simulink model "Experiment_06081908_cs"  (R2021a)
settings: Solver=ode5  StartTime=0.0  StopTime=30  FixedStep=1/1000  RelTol=1e-3
PreLoadFcn:
  | mbxruntime.callbacks.PreLoadFcn(bdroot);
PostLoadFcn:
  | mbxruntime.callbacks.PostLoadFcn(bdroot);
InitFcn:
  | mbxruntime.callbacks.InitFcn(bdroot);
StartFcn:
  | mbxruntime.callbacks.StartFcn(bdroot);
StopFcn:
  | mbxruntime.callbacks.StopFcn(bdroot);
model workspace (MAT data in the model file):
  mbox_table : object (value not decoded)
  model_closed = 0
  sim_status = 0
values from neighbouring files (symbols this model uses):
  c_factor = 43.75    [emplanner_init.m]
  cf = -175016    [emplanner_init.m]
  cr = -130634    [emplanner_init.m]
  KD_PID_distance = 0.0    (= 0)    [emplanner_init.m]
  KD_PID_speed = 0    [emplanner_init.m]
  KI_PID_distance = 0.0    (= 0)    [emplanner_init.m]
  KI_PID_speed = 0    [emplanner_init.m]
  KP_PID_distance = 0.5    [emplanner_init.m]
  KP_PID_speed = 1.8    [emplanner_init.m]
  la = 1.265    [emplanner_init.m]
  lb = 2.947-1.265    (= 1.682)    [emplanner_init.m]
  LQR_K1 = k(:,1)'    [emplanner_init.m]
  LQR_K2 = k(:,2)'    [emplanner_init.m]
  LQR_K3 = k(:,3)'    [emplanner_init.m]
  LQR_K4 = k(:,4)'    [emplanner_init.m]
  m = 2020    [emplanner_init.m]
  rack_displacement = [-39.14 , -37.2 , -35.29 , -33.43 , -31.6 , -29.81 , -28.06 , -26.34 , -24.66 ,      -23.01 , -21.38 , -19.79 , -18.23 , -16.69 , -15.18 , -13.7 , -12.23 , -10.8 , -9.38 , -7.98 ,     -6.61 , -5.25 , -3.91 , -2.59 , -1.29 , 0 , 1.27 , 2.54 , 3.78 , 5.02 , 6.24 , 7.46 , 8.66 ,      9.86 , 11.05 , 12.24 , 13.41 , 14.59 , 15.76 , 16.92 , 18.09 , 19.25 , 20.42 , 21.59 , 22.76 ,      23.93 , 25.11 , 26 ...(+26 chars)    [emplanner_init.m]
  right_wheel_ground = [-70 ,-67.2 , -64.4 , -61.6 , -58.8 , -56 , -53.2 , -50.4 , -47.6 , -44.8 , -42 ,      -39.2 , -36.4 , -33.6 , -30.8 , -28 , -25.2 , -22.4 , -19.6 , -16.8 , -14 , -11.2 , -8.4 , -5.6 ,      -2.8 , 0 , 2.8 , 5.6 , 8.4 , 11.2 , 14 , 16.8 , 19.6 , 22.4 , 25.2 , 28 , 30.8 , 33.6 , 36.4 ,      39.2 , 42 , 44.8 , 47.6 , 50.4 , 53.2 , 56 , 58.8 , 61.6 , 64.4 , 67.2 , 70 ]    [emplanner_init.m]
  vx_break_point = zeros(1,5000)    [emplanner_init.m]
undefined symbols (not defined in the file or in its folder): aubr, DiscIntNeverNeededParam, global_path_x, global_path_y, tablebr, vubr
libraries: PreScanSimulinkLibrary x18, Solver_SF x1, simulink_extras x1
(part 4 of 8)

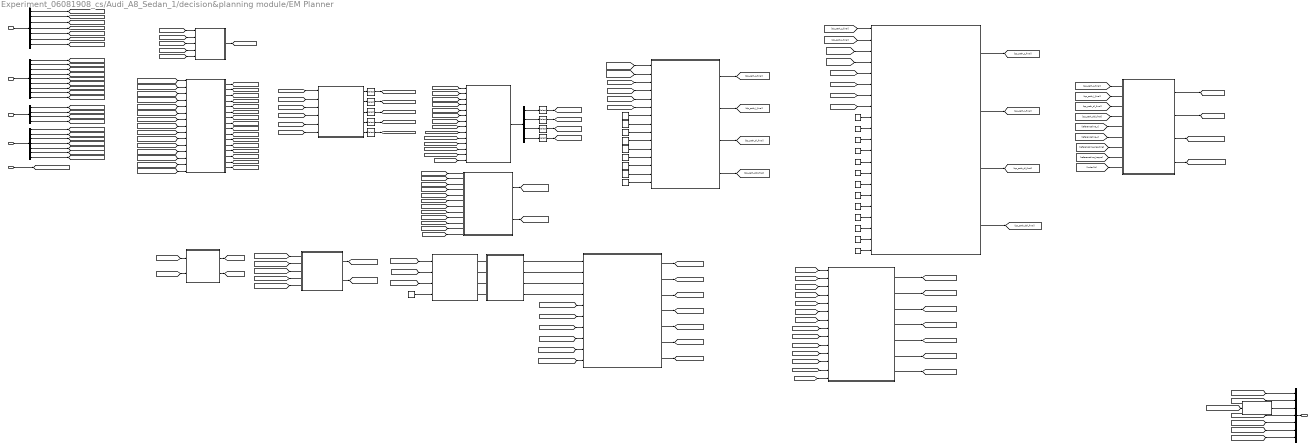
== system Experiment_06081908_cs/Audi_A8_Sedan_1/decision&planning module/EM Planner ==
  referenceline info : Inport
  location info : Inport  Port=2
  perception info : Inport  Port=3
  pre_planning info : Inport  Port=4
  current time : Inport  Port=5
  Bus Creator : BusCreator  Inputs=7
  Bus Selector : BusSelector  OutputSignals=referenceline_x,referenceline_y,referenceline_heading,referenceline_kappa,origin_match_point_index,origin_x,origin_y
  Bus Selector1 : BusSelector  OutputSignals=host_x,host_y,host_heading_xy,host_vx,host_vy,host_yawrate,host_speed,host_ax,host_ay
  Bus Selector2 : BusSelector  OutputSignals=obs_x_set_gcs,obs_y_set_gcs,obs_velocity_set_gcs,obs_heading_set_gcs
  Bus Selector3 : BusSelector  OutputSignals=trajectory_x_gcs,trajectory_y_gcs,trajectory_heading_gcs,trajectory_kappa_gcs,trajectory_speed_gcs,trajectory_accel_gcs,trajectory_time_gcs
  Bus Selector4 : BusSelector  OutputSignals=s_set,l_set,dl_set,ddl_set
  Cartesian2Frenet : Subsystem
  Constant : Constant  Value=1e6
  Constant1 : Constant  Value=2000
  Constant10 : Constant  Value=0.1
  Constant11 : Constant  Value=0.02
  Constant12 : Constant  Value=2
  Constant13 : Constant  Value=25000
  Constant14 : Constant  Value=50
  Constant15 : Constant  Value=20
  Constant{7,16..19} (5 alike) : Constant  Value=15
  Constant2 : Constant  Value=2
  Constant20 : Constant  Value=3
  Constant21 : Constant  Value=3
  Constant22 : Constant  Value=1.63
  Constant3 : Constant  Value=3
  Constant4 : Constant  Value=10
  Constant5 : Constant  Value=11
  Constant6 : Constant  Value=4
  Constant8 : Constant
  Constant9 : Constant  Value=6
  Frenet2Cartesian task : MATLAB Function  TreatAsAtomicUnit=on
  MATLAB Function : MATLAB Function  TreatAsAtomicUnit=on
  MATLAB Function2 : MATLAB Function  TreatAsAtomicUnit=on
  Selector{1..9} (9 alike) : Selector  InputPortWidth=128  IndexOptions=Index vector (dialog)  Indices=1  OutputSizes=1
  calc path length and map between point and s : MATLAB Function  TreatAsAtomicUnit=on
  calc plan start info and stitch trajectory : MATLAB Function  TreatAsAtomicUnit=on
  calc speed planning start condition : MATLAB Function  TreatAsAtomicUnit=on
  genrate index to s : MATLAB Function  TreatAsAtomicUnit=on
  increase st point count : MATLAB Function  TreatAsAtomicUnit=on
  obs : Subsystem
  path and speed merge : MATLAB Function  TreatAsAtomicUnit=on
  path decision task : Subsystem
  path planning task : Subsystem
  simple speed qp planning : MATLAB Function  TreatAsAtomicUnit=on
  stitch trajectory : MATLAB Function  TreatAsAtomicUnit=on
  EM Planner result : Outport
  wires:
  referenceline info/1 -> Bus Selector/1
  location info/1 -> Bus Selector1/1
  perception info/1 -> Bus Selector2/1
  pre_planning info/1 -> Bus Selector3/1
  current time/1 -> [current_time]
  Bus Selector3/1 -> [pre_trajectory_x_gcs]  "<trajectory_x_gcs>"
  Bus Selector3/2 -> [pre_trajectory_y_gcs]  "<trajectory_y_gcs>"
  Bus Selector3/3 -> [pre_trajectory_heading_gcs]  "<trajectory_heading_gcs>"
  Bus Selector3/4 -> [pre_trajectory_kappa_gcs]  "<trajectory_kappa_gcs>"
  Bus Selector3/5 -> [pre_trajectory_speed_gcs]  "<trajectory_speed_gcs>"
  Bus Selector3/6 -> [pre_trajectory_accel_gcs]  "<trajectory_accel_gcs>"
  Bus Selector3/7 -> [pre_trajectory_time]  "<trajectory_time_gcs>"
  Bus Selector2/1 -> [obs_x_set_gcs]  "<obs_x_set_gcs>"
  Bus Selector2/2 -> [obs_y_set_gcs]  "<obs_y_set_gcs>"
  Bus Selector2/3 -> [obs_velocity_set_gcs]  "<obs_velocity_set_gcs>"
  Bus Selector2/4 -> [obs_heading_set_gcs]  "<obs_heading_set_gcs>"
  Bus Selector1/1 -> [host_x]  "<host_x>"
  Bus Selector1/2 -> [host_y]  "<host_y>"
  Bus Selector1/3 -> [host_heading_xy]  "<host_heading_xy>"
  Bus Selector1/4 -> [host_vx_vcs]  "<host_vx>"
  Bus Selector1/5 -> [host_vy_vcs]  "<host_vy>"
  Bus Selector1/6 -> [host_yawrate]  "<host_yawrate>"
  Bus Selector1/7 -> [host_speed]  "<host_speed>"
  Bus Selector1/8 -> [host_ax_vcs]  "<host_ax>"
  Bus Selector1/9 -> [host_ay_vcs]  "<host_ay>"
  Bus Selector/1 -> [referenceline_x]  "<referenceline_x>"
  Bus Selector/2 -> [referenceline_y]  "<referenceline_y>"
  Bus Selector/3 -> [referenceline_heading]  "<referenceline_heading>"
  Bus Selector/4 -> [referenceline_kappa]  "<referenceline_kappa>"
  [host_ay_vcs] -> calc plan start info and stitch trajectory/15(host_ay)
  [host_ax_vcs] -> calc plan start info and stitch trajectory/14(host_ax)
  [host_vy_vcs] -> calc plan start info and stitch trajectory/13(host_vy)
  [host_vx_vcs] -> calc plan start info and stitch trajectory/12(host_vx)
  [host_heading_xy] -> calc plan start info and stitch trajectory/11(host_heading_xy)
  [host_y] -> calc plan start info and stitch trajectory/10(host_y)
  [host_x] -> calc plan start info and stitch trajectory/9(host_x)
  [current_time] -> calc plan start info and stitch trajectory/8(current_time)
  [pre_trajectory_x_gcs] -> calc plan start info and stitch trajectory/1(pre_trajectory_x)
  [pre_trajectory_y_gcs] -> calc plan start info and stitch trajectory/2(pre_trajectory_y)
  [pre_trajectory_time] -> calc plan start info and stitch trajectory/7(pre_trajectory_time)
  [pre_trajectory_accel_gcs] -> calc plan start info and stitch trajectory/6(pre_trajectory_accel)
  [pre_trajectory_speed_gcs] -> calc plan start info and stitch trajectory/5(pre_trajectory_velocity)
  [pre_trajectory_kappa_gcs] -> calc plan start info and stitch trajectory/4(pre_trajectory_kappa)
  [pre_trajectory_heading_gcs] -> calc plan start info and stitch trajectory/3(pre_trajectory_heading)
  calc plan start info and stitch trajectory/1(plan_start_x) -> [plan_start_x_gcs]
  calc plan start info and stitch trajectory/2(plan_start_y) -> [plan_start_y_gcs]
  calc plan start info and stitch trajectory/3(plan_start_heading) -> [plan_start_heading_gcs]
  calc plan start info and stitch trajectory/4(plan_start_kappa) -> [plan_start_kappa_gcs]
  calc plan start info and stitch trajectory/5(plan_start_vx) -> [plan_start_vx_gcs]
  calc plan start info and stitch trajectory/6(plan_start_vy) -> [plan_start_vy_gcs]
  calc plan start info and stitch trajectory/7(plan_start_ax) -> [plan_start_ax_gcs]
  calc plan start info and stitch trajectory/8(plan_start_ay) -> [plan_start_ay_gcs]
  calc plan start info and stitch trajectory/9(plan_start_time) -> [plan_start_time]
  calc plan start info and stitch trajectory/10(stitch_x) -> [stitch_x_gcs]
  calc plan start info and stitch trajectory/11(stitch_y) -> [stitch_y_gcs]
  calc plan start info and stitch trajectory/12(stitch_heading) -> [stitch_heading_gcs]
  calc plan start info and stitch trajectory/13(stitch_kappa) -> [stitch_kappa_gcs]
  calc plan start info and stitch trajectory/14(stitch_speed) -> [stitch_speed_gcs]
  calc plan start info and stitch trajectory/15(stitch_accel) -> [stitch_accel_gcs]
  calc plan start info and stitch trajectory/16(stitch_time) -> [stitch_time]
  Bus Selector/5 -> [origin_match_point_index]  "<origin_match_point_index>"
  Bus Selector/6 -> [origin_x]  "<origin_x>"
  Bus Selector/7 -> [origin_y]  "<origin_y>"
  [referenceline_x] -> genrate index to s/1(path_x)
  [referenceline_y] -> genrate index to s/2(path_y)
  [origin_x] -> genrate index to s/3(origin_x)
  [origin_y] -> genrate index to s/4(origin_y)
  [origin_match_point_index] -> genrate index to s/5(origin_match_point_index)
  genrate index to s/1(index2s) -> [index2s]
  MATLAB Function2/5(proj_kappa_set) -> Selector5/1
  MATLAB Function2/3(proj_y_set) -> Selector3/1
  MATLAB Function2/1(match_point_index_set) -> Selector1/1
  MATLAB Function2/4(proj_heading_set) -> Selector4/1
  MATLAB Function2/2(proj_x_set) -> Selector2/1
  [plan_start_x_gcs] -> MATLAB Function2/1(x_set)
  [plan_start_y_gcs] -> MATLAB Function2/2(y_set)
  [referenceline_x] -> MATLAB Function2/3(frenet_path_x)
  [referenceline_y] -> MATLAB Function2/4(frenet_path_y)
  [referenceline_heading] -> MATLAB Function2/5(frenet_path_heading)
  [referenceline_kappa] -> MATLAB Function2/6(frenet_path_kappa)
  Selector1/1 -> [plan_start_match_point_index]
  Selector2/1 -> [plan_start_proj_x]
  Selector3/1 -> [plan_start_proj_y]
  Selector4/1 -> [plan_start_proj_heading]
  Selector5/1 -> [plan_start_proj_kappa]
  [plan_start_y_gcs] -> Cartesian2Frenet/2(y_set)
  [plan_start_x_gcs] -> Cartesian2Frenet/1(x_set)
  [plan_start_vx_gcs] -> Cartesian2Frenet/3(vx_set)
  [plan_start_vy_gcs] -> Cartesian2Frenet/4(vy_set)
  [plan_start_ax_gcs] -> Cartesian2Frenet/5(ax_set)
  [plan_start_ay_gcs] -> Cartesian2Frenet/6(ay_set)
  [referenceline_x] -> Cartesian2Frenet/7(frenet_path_x)
  [referenceline_y] -> Cartesian2Frenet/8(frenet_path_y)
  [plan_start_match_point_index] -> Cartesian2Frenet/9(proj_match_point_index_set)
  [plan_start_proj_x] -> Cartesian2Frenet/10(proj_x_set)
  [plan_start_proj_y] -> Cartesian2Frenet/11(proj_y_set)
  [plan_start_proj_heading] -> Cartesian2Frenet/12(proj_heading_set)
  [plan_start_proj_kappa] -> Cartesian2Frenet/13(proj_kappa_set)
  Cartesian2Frenet/1(Cartesian2FrenetOut) -> Bus Selector4/1
  Bus Selector4/4 -> Selector9/1  "<ddl_set>"
  Bus Selector4/3 -> Selector8/1  "<dl_set>"
  Bus Selector4/2 -> Selector7/1  "<l_set>"
  Bus Selector4/1 -> Selector6/1  "<s_set>"
  Selector6/1 -> [plan_start_s]
  Selector7/1 -> [plan_start_l]
  Selector8/1 -> [plan_start_dl]
  Selector9/1 -> [plan_start_ddl]
  [index2s] -> Cartesian2Frenet/14(index2s)
  [host_x] -> obs/1(host_x)
  [host_y] -> obs/2(host_y)
  [host_heading_xy] -> obs/3(host_heading_xy)
  [obs_x_set_gcs] -> obs/4(obs_x_set_gcs)
  [obs_y_set_gcs] -> obs/5(obs_y_set_gcs)
  [obs_velocity_set_gcs] -> obs/6(obs_velocity_set_gcs)
  [obs_heading_set_gcs] -> obs/7(obs_heading_set_gcs)
  [referenceline_x] -> obs/8(referenceline_x)
  [referenceline_y] -> obs/9(referenceline_y)
  [referenceline_heading] -> obs/10(referenceline_heading)
  [referenceline_kappa] -> obs/11(referenceline_kappa)
  [index2s] -> obs/12(index2s)
  obs/1(static_obs_s_set) -> [static_obs_s_set]
  obs/2(static_obs_l_set) -> [static_obs_l_set]
  path and speed merge/7(trajectory_time) -> [trajectory_time]
  path and speed merge/1(trajectory_x) -> [trajectory_x]
  [trajectory_speed] -> stitch trajectory/5(trajectory_speed)
  path and speed merge/4(trajectory_kappa) -> [trajectory_kappa]
  [plan_start_vy_gcs] -> calc speed planning start condition/2(plan_start_vy)
  [stitch_time] -> stitch trajectory/14(stitch_time)
  calc path length and map between point and s/2(path_s) -> [path_s]
  [plan_start_heading_gcs] -> calc speed planning start condition/5(plan_start_heading)
  simple speed qp planning/2(s_dot_init) -> increase st point count/2(s_dot_init)
  Bus Creator/1 -> EM Planner result/1
  simple speed qp planning/1(s_init) -> increase st point count/1(s_init)
  [trajectory_x_final] -> Bus Creator/1  "trajectory_x_gcs"
  stitch trajectory/4(trajectory_kappa_final) -> [trajectory_kappa_final]
  [plan_start_ax_gcs] -> calc speed planning start condition/3(plan_start_ax)
  calc speed planning start condition/1(plan_start_s_dot) -> [plan_start_s_dot]
  [plan_start_ay_gcs] -> calc speed planning start condition/4(plan_start_ay)
  [stitch_speed_gcs] -> stitch trajectory/12(stitch_speed)
  [trajectory_time_final] -> Bus Creator/7  "trajectory_time_gcs"
  Constant9/1 -> simple speed qp planning/4(recommend_T)
  [stitch_x_gcs] -> stitch trajectory/8(stitch_x)
  stitch trajectory/1(trajectory_x_final) -> [trajectory_x_final]
  [trajectory_accel_final] -> Bus Creator/6  "trajectory_accel_gcs"
  [stitch_heading_gcs] -> stitch trajectory/10(stitch_heading)
  [trajectory_speed_final] -> Bus Creator/5  "trajectory_speed_gcs"
  [stitch_y_gcs] -> stitch trajectory/9(stitch_y)
  stitch trajectory/6(trajectory_accel_final) -> [trajectory_accel_final]
  [plan_start_s_dot2] -> simple speed qp planning/2(plan_start_s_dot2)
  increase st point count/3(s_dot2) -> path and speed merge/3(s_dot2)
  [plan_start_vx_gcs] -> calc speed planning start condition/1(plan_start_vx)
  [trajectory_heading_final] -> MATLAB Function/1(trajectory_heading_final)
  [trajectory_accel] -> stitch trajectory/6(trajectory_accel)
  [trajectory_kappa] -> stitch trajectory/4(trajectory_kappa)
  stitch trajectory/7(trajectory_time_final) -> [trajectory_time_final]
  [trajectory_x_init] -> path and speed merge/7(trajectory_x_init)
  stitch trajectory/2(trajectory_y_final) -> [trajectory_y_final]
  increase st point count/2(s_dot) -> path and speed merge/2(s_dot)
  stitch trajectory/3(trajectory_heading_final) -> [trajectory_heading_final]
  [trajectory_kappa_final] -> Bus Creator/4  "trajectory_kappa_gcs"
  [plan_start_s_dot] -> simple speed qp planning/1(plan_start_s_dot)
  path and speed merge/3(trajectory_heading) -> [trajectory_heading]
  simple speed qp planning/3(s_dot2_init) -> increase st point count/3(s_dot2_init)
  stitch trajectory/5(trajectory_speed_final) -> [trajectory_speed_final]
  [trajectory_y_final] -> Bus Creator/2  "trajectory_y_gcs"
  [trajectory_y] -> stitch trajectory/2(trajectory_y)
  calc path length and map between point and s/1(path_s_end) -> [path_s_end]
  calc speed planning start condition/2(plan_start_s_dot2) -> [plan_start_s_dot2]
  [trajectory_kappa_init] -> path and speed merge/10(trajectory_kappa_init)
  [stitch_accel_gcs] -> stitch trajectory/13(stitch_accel)
  increase st point count/1(s) -> path and speed merge/1(s)
  [trajectory_x] -> stitch trajectory/1(trajectory_x)
  [trajectory_y_init] -> calc path length and map between point and s/2(trajectory_y)
  [path_s_end] -> simple speed qp planning/3(s_end)
  path and speed merge/6(trajectory_accel) -> [trajectory_accel]
  [stitch_kappa_gcs] -> stitch trajectory/11(stitch_kappa)
  increase st point count/4(relative_time) -> path and speed merge/4(relative_time)
  [path_s] -> path and speed merge/6(path_s)
  path and speed merge/2(trajectory_y) -> [trajectory_y]
  [trajectory_heading_init] -> path and speed merge/9(trajectory_heading_init)
  [plan_start_time] -> path and speed merge/5(current_time)
  path and speed merge/5(trajectory_speed) -> [trajectory_speed]
  simple speed qp planning/4(relative_time_init) -> increase st point count/4(relative_time_init)
  [trajectory_y_init] -> path and speed merge/8(trajectory_y_init)
  [trajectory_time] -> stitch trajectory/7(trajectory_time)
  [trajectory_heading] -> stitch trajectory/3(trajectory_heading)
  [trajectory_x_init] -> calc path length and map between point and s/1(trajectory_x)
  [index2s] -> Frenet2Cartesian task/9(index2s)
  [referenceline_x] -> Frenet2Cartesian task/5(frenet_path_x)
  [referenceline_y] -> Frenet2Cartesian task/6(frenet_path_y)
  [referenceline_heading] -> Frenet2Cartesian task/7(frenet_path_heading)
  [referenceline_kappa] -> Frenet2Cartesian task/8(frenet_path_kappa)
  Frenet2Cartesian task/1(x_set) -> [trajectory_x_init]
  Frenet2Cartesian task/2(y_set) -> [trajectory_y_init]
  Frenet2Cartesian task/3(heading_set) -> [trajectory_heading_init]
  Frenet2Cartesian task/4(kappa_set) -> [trajectory_kappa_init]
  path decision task/1(dp_path_s_final) -> [dp_path_s_final]
  path decision task/2(dp_path_l_final) -> [dp_path_l_final]
  path decision task/3(dp_path_dl_final) -> [dp_path_dl_final]
  path decision task/4(dp_path_ddl_final) -> [dp_path_ddl_final]
  [static_obs_s_set] -> path decision task/1(static_obs_s_set)
  [static_obs_l_set] -> path decision task/2(static_obs_l_set)
  [plan_start_ddl] -> path decision task/6(plan_start_ddl)
  [plan_start_dl] -> path decision task/5(plan_start_dl)
  [plan_start_l] -> path decision task/4(plan_start_l)
  [plan_start_s] -> path decision task/3(plan_start_s)
  [dp_path_s_final] -> path planning task/1(dp_path_s_final)
  [dp_path_l_final] -> path planning task/2(dp_path_l_final)
  [plan_start_l] -> path planning task/6(plan_start_l)
  [plan_start_ddl] -> path planning task/8(plan_start_ddl)
  [plan_start_dl] -> path planning task/7(plan_start_dl)
  Constant22/1 -> path planning task/19(host_w)
  Constant21/1 -> path planning task/18(host_d2)
  Constant20/1 -> path planning task/17(host_d1)
  Constant19/1 -> path planning task/16(qp_cost_end_ddl)
  Constant18/1 -> path planning task/15(qp_cost_end_dl)
  Constant17/1 -> path planning task/14(qp_cost_endl)
  Constant16/1 -> path planning task/13(qp_cost_centre)
  Constant15/1 -> path planning task/12(qp_cost_dddl)
  Constant14/1 -> path planning task/11(qp_cost_ddl)
  Constant13/1 -> path planning task/10(qp_cost_dl)
  Constant12/1 -> path planning task/9(qp_cost_l)
  Constant8/1 -> path decision task/15(dp_sample_l)
  Constant7/1 -> path decision task/14(dp_sample_s)
  Constant6/1 -> path decision task/13(dp_col)
  Constant5/1 -> path decision task/12(dp_row)
  Constant4/1 -> path decision task/11(dp_cost_ref)
  Constant3/1 -> path decision task/10(dp_cost_dddl)
  Constant/1 -> path decision task/7(dp_cost_collision)
  Constant1/1 -> path decision task/8(dp_cost_dl)
  Constant2/1 -> path decision task/9(dp_cost_ddl)
  [static_obs_s_set] -> path planning task/3(static_obs_s_set)
  [static_obs_l_set] -> path planning task/4(static_obs_l_set)
  Constant10/1 -> path planning task/20(delta_dl_max)
  Constant11/1 -> path planning task/21(delta_ddl_max)
  path planning task/1(qp_path_s_final) -> [qp_path_s_final]
  path planning task/2(qp_path_l_final) -> [qp_path_l_final]
  path planning task/3(qp_path_dl_final) -> [qp_path_dl_final]
  path planning task/4(qp_path_ddl_final) -> [qp_path_ddl_final]
  [qp_path_ddl_final] -> Frenet2Cartesian task/4(ddl_set)
  [qp_path_l_final] -> Frenet2Cartesian task/2(l_set)
  [qp_path_dl_final] -> Frenet2Cartesian task/3(dl_set)
  [qp_path_s_final] -> Frenet2Cartesian task/1(s_set)
  [plan_start_s] -> path planning task/5(plan_start_s)
  MATLAB Function/1(y) -> Bus Creator/3  "trajectory_heading_gcs"

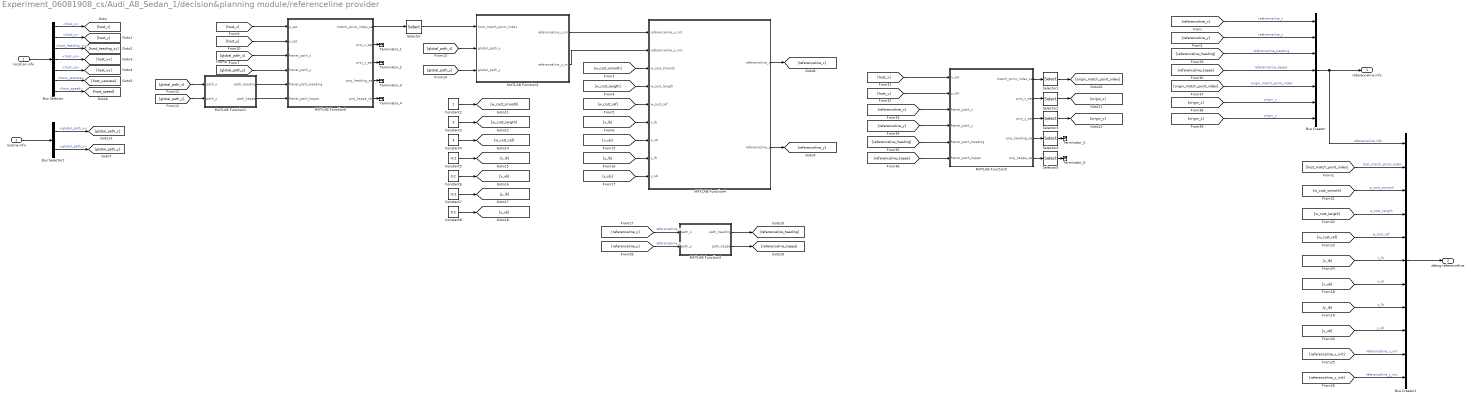
== system Experiment_06081908_cs/Audi_A8_Sedan_1/decision&planning module/referenceline provider ==
  location info : Inport
  routine info : Inport  Port=2
  Bus Creator : BusCreator  Inputs=7
  Bus Creator1 : BusCreator  Inputs=11
  Bus Selector : BusSelector  OutputSignals=host_x,host_y,host_heading_xy,host_vx,host_vy,host_yawrate,host_speed
  Bus Selector1 : BusSelector  OutputSignals=global_path_x,global_path_y
  Constant2 : Constant
  Constant3 : Constant  Value=2
  Constant4 : Constant  Value=3
  Constant5 : Constant  Value=-0.2
  Constant6 : Constant  Value=0.2
  Constant7 : Constant  Value=-0.2
  Constant8 : Constant  Value=0.2
  MATLAB Function1 : MATLAB Function  TreatAsAtomicUnit=on
  MATLAB Function2 : MATLAB Function  TreatAsAtomicUnit=on
  MATLAB Function3 : MATLAB Function  TreatAsAtomicUnit=on
  MATLAB Function4 : MATLAB Function  TreatAsAtomicUnit=on
  MATLAB Function5 : MATLAB Function  TreatAsAtomicUnit=on
  MATLAB Function6 : MATLAB Function  TreatAsAtomicUnit=on
  Selector{,1..5} (6 alike) : Selector  InputPortWidth=128  IndexOptions=Index vector (dialog)  Indices=1  OutputSizes=1
  Terminator_{1..6} (6 alike) : Terminator
  referenceline info : Outport
  debug referenceline : Outport  Port=2
  wires:
  [global_path_x] -> MATLAB Function2/2(global_path_x)
  [host_x] -> MATLAB Function6/1(x_set)
  MATLAB Function1/2(path_kappa) -> MATLAB Function6/6(frenet_path_kappa)
  MATLAB Function1/1(path_heading) -> MATLAB Function6/5(frenet_path_heading)
  [global_path_y] -> MATLAB Function6/4(frenet_path_y)
  [global_path_x] -> MATLAB Function6/3(frenet_path_x)
  [host_y] -> MATLAB Function6/2(y_set)
  [global_path_y] -> MATLAB Function1/2(path_y)
  [global_path_x] -> MATLAB Function1/1(path_x)
  Selector/1 -> MATLAB Function2/1(host_match_point_index)
  MATLAB Function6/1(match_point_index_set) -> Selector/1
  [global_path_y] -> MATLAB Function2/3(global_path_y)
  MATLAB Function2/1(referenceline_x_init) -> MATLAB Function4/1(referenceline_x_init)
  Bus Selector/5 -> [host_vy]  "<host_vy>"
  Bus Selector/1 -> [host_x]  "<host_x>"
  Bus Selector/2 -> [host_y]  "<host_y>"
  Bus Selector/3 -> [host_heading_xy]  "<host_heading_xy>"
  Bus Selector/4 -> [host_vx]  "<host_vx>"
  Bus Selector/7 -> [host_speed]  "<host_speed>"
  Bus Selector/6 -> [host_yawrate]  "<host_yawrate>"
  location info/1 -> Bus Selector/1
  Bus Selector1/2 -> [global_path_y]  "<global_path_y>"
  Bus Selector1/1 -> [global_path_x]  "<global_path_x>"
  routine info/1 -> Bus Selector1/1
  MATLAB Function4/1(referenceline_x) -> [referenceline_x]
  MATLAB Function4/2(referenceline_y) -> [referenceline_y]
  [referenceline_x] -> Bus Creator/1  "referenceline_x"
  [referenceline_y] -> Bus Creator/2  "referenceline_y"
  Bus Creator1/1 -> debug referenceline/1
  Bus Creator/1 -> Bus Creator1/1, referenceline info/1  "referenceline info"
  Constant2/1 -> [w_cost_smooth]
  Constant3/1 -> [w_cost_length]
  Constant8/1 -> [y_ub]
  Constant7/1 -> [y_lb]
  Constant6/1 -> [x_ub]
  Constant5/1 -> [x_lb]
  Constant4/1 -> [w_cost_ref]
  [w_cost_smooth] -> MATLAB Function4/3(w_cost_smooth)
  [w_cost_length] -> MATLAB Function4/4(w_cost_length)
  [w_cost_ref] -> MATLAB Function4/5(w_cost_ref)
  [x_lb] -> MATLAB Function4/6(x_lb)
  [x_ub] -> MATLAB Function4/7(x_ub)
  [y_lb] -> MATLAB Function4/8(y_lb)
  [y_ub] -> MATLAB Function4/9(y_ub)
  MATLAB Function2/2(referenceline_y_init) -> MATLAB Function4/2(referenceline_y_init)
  [w_cost_ref] -> Bus Creator1/5  "w_cost_ref"
  [x_lb] -> Bus Creator1/6  "x_lb"
  [w_cost_length] -> Bus Creator1/4  "w_cost_length"
  [x_ub] -> Bus Creator1/7  "x_ub"
  [w_cost_smooth] -> Bus Creator1/3  "w_cost_smooth"
  [y_lb] -> Bus Creator1/8  "y_lb"
  [host_match_point_index] -> Bus Creator1/2  "host_match_point_index"
  [y_ub] -> Bus Creator1/9  "y_ub"
  [referenceline_x_init] -> Bus Creator1/10  "referenceline_x_init"
  [referenceline_y_init] -> Bus Creator1/11  "referenceline_y_init"
  [referenceline_x] -> MATLAB Function3/1(path_x)  "referenceline_x"
  [referenceline_y] -> MATLAB Function3/2(path_y)  "referenceline_y"
  MATLAB Function3/1(path_heading) -> [referenceline_heading]
  MATLAB Function3/2(path_kappa) -> [referenceline_kappa]
  [referenceline_kappa] -> Bus Creator/4  "referenceline_kappa"
  [referenceline_heading] -> Bus Creator/3  "referenceline_heading"
  [host_x] -> MATLAB Function5/1(x_set)
  [host_y] -> MATLAB Function5/2(y_set)
  [referenceline_x] -> MATLAB Function5/3(frenet_path_x)
  [referenceline_y] -> MATLAB Function5/4(frenet_path_y)
  [referenceline_heading] -> MATLAB Function5/5(frenet_path_heading)
  [referenceline_kappa] -> MATLAB Function5/6(frenet_path_kappa)
  MATLAB Function5/1(match_point_index_set) -> Selector1/1
  MATLAB Function5/2(proj_x_set) -> Selector2/1
  MATLAB Function5/3(proj_y_set) -> Selector3/1
  MATLAB Function5/4(proj_heading_set) -> Selector4/1
  MATLAB Function5/5(proj_kappa_set) -> Selector5/1
  Selector1/1 -> [origin_match_point_index]
  Selector2/1 -> [origin_x]
  Selector3/1 -> [origin_y]
  [origin_match_point_index] -> Bus Creator/5  "origin_match_point_index"
  [origin_x] -> Bus Creator/6  "origin_x"
  [origin_y] -> Bus Creator/7  "origin_y"
  MATLAB Function6/2(proj_x_set) -> Terminator_1/1
  MATLAB Function6/3(proj_y_set) -> Terminator_2/1
  MATLAB Function6/4(proj_heading_set) -> Terminator_3/1
  MATLAB Function6/5(proj_kappa_set) -> Terminator_4/1
  Selector4/1 -> Terminator_5/1
  Selector5/1 -> Terminator_6/1

== system Experiment_06081908_cs/Audi_A8_Sedan_2/SELF_Demux/compas converter ==
  rotz [rad] : Inport
  cart2compas : Subsystem
  rad2deg : Gain  Gain=180/pi
  heading [deg] : Outport
  wires:
  rad2deg/1 -> cart2compas/1(Angle [deg])
  rotz [rad]/1 -> rad2deg/1
  cart2compas/1(heading [deg]) -> heading [deg]/1

== system Experiment_06081908_cs/Audi_A8_Sedan_2/Trajectories/Traj2State1 ==
  Traj Org : Inport
  Offset : Inport  Port=2
  Add2 : Sum
  ApplyRotation : PreScanSimulinkLibrary/ApplyRotation  SystemSampleTime=-1  VariantActivationTime=update diagram  Latency=0  AutoFrameSizeCalculation=off
  ApplyRotation1 : PreScanSimulinkLibrary/ApplyRotation  SystemSampleTime=-1  VariantActivationTime=update diagram  Latency=0  AutoFrameSizeCalculation=off
  ApplyRotation2 : PreScanSimulinkLibrary/ApplyRotation  SystemSampleTime=-1  VariantActivationTime=update diagram  Latency=0  AutoFrameSizeCalculation=off
  Constant : Constant  Value=zeros(12,1)
  Mux : Mux  Inputs=6
  Mux1 : Mux  Inputs=2
  Mux{2,4..9} (7 alike) : Mux  Inputs=3
  Mux3 : Mux  Inputs=2
  Selector : Selector  InputPortWidth=6  IndexOptions=Index vector (dialog)  Indices=[4 5 6]  OutputSizes=1
  Selector1 : Selector  InputPortWidth=21  IndexOptions=Index vector (dialog)  Indices=[5]  OutputSizes=1
  Selector10 : Selector  InputPortWidth=21  IndexOptions=Index vector (dialog)  Indices=[2]  OutputSizes=1
  Selector11 : Selector  InputPortWidth=21  IndexOptions=Index vector (dialog)  Indices=[3]  OutputSizes=1
  Selector12 : Selector  InputPortWidth=21  IndexOptions=Index vector (dialog)  Indices=[1]  OutputSizes=1
  Selector13 : Selector  InputPortWidth=21  IndexOptions=Index vector (dialog)  Indices=[8]  OutputSizes=1
  Selector14 : Selector  InputPortWidth=21  IndexOptions=Index vector (dialog)  Indices=[9]  OutputSizes=1
  Selector15 : Selector  InputPortWidth=21  IndexOptions=Index vector (dialog)  Indices=[7]  OutputSizes=1
  Selector16 : Selector  InputPortWidth=21  IndexOptions=Index vector (dialog)  Indices=[14]  OutputSizes=1
  Selector17 : Selector  InputPortWidth=21  IndexOptions=Index vector (dialog)  Indices=[15]  OutputSizes=1
  Selector18 : Selector  InputPortWidth=21  IndexOptions=Index vector (dialog)  Indices=[13]  OutputSizes=1
  Selector19 : Selector  InputPortWidth=21  IndexOptions=Index vector (dialog)  Indices=[20]  OutputSizes=1
  Selector2 : Selector  InputPortWidth=21  IndexOptions=Index vector (dialog)  Indices=[6]  OutputSizes=1
  Selector20 : Selector  InputPortWidth=21  IndexOptions=Index vector (dialog)  Indices=[21]  OutputSizes=1
  Selector21 : Selector  InputPortWidth=21  IndexOptions=Index vector (dialog)  Indices=[19]  OutputSizes=1
  Selector3 : Selector  InputPortWidth=21  IndexOptions=Index vector (dialog)  Indices=[12]  OutputSizes=1
  Selector4 : Selector  InputPortWidth=21  IndexOptions=Index vector (dialog)  Indices=[17]  OutputSizes=1
  Selector5 : Selector  InputPortWidth=21  IndexOptions=Index vector (dialog)  Indices=[18]  OutputSizes=1
  Selector6 : Selector  InputPortWidth=21  IndexOptions=Index vector (dialog)  Indices=[16]  OutputSizes=1
  Selector7 : Selector  InputPortWidth=21  IndexOptions=Index vector (dialog)  Indices=[11]  OutputSizes=1
  Selector8 : Selector  InputPortWidth=21  IndexOptions=Index vector (dialog)  Indices=[10]  OutputSizes=1
  Selector9 : Selector  InputPortWidth=21  IndexOptions=Index vector (dialog)  Indices=[4]  OutputSizes=1
  Traj2State2 : Subsystem
  state : Outport
  wires:
  Mux9/1 -> ApplyRotation2/2, ApplyRotation1/2, ApplyRotation/2
  Selector20/1 -> Mux9/3
  Selector19/1 -> Mux9/2
  Selector21/1 -> Mux9/1
  Selector5/1 -> Mux8/3
  Selector4/1 -> Mux8/2
  Selector6/1 -> Mux8/1
  Mux8/1 -> Mux/6
  Mux6/1 -> ApplyRotation2/1
  Mux7/1 -> Mux/4
  ApplyRotation2/1 -> Mux/5
  Selector3/1 -> Mux7/3
  Selector7/1 -> Mux7/2
  Selector8/1 -> Mux7/1
  Mux4/1 -> Mux/2
  Mux5/1 -> ApplyRotation1/1
  ApplyRotation1/1 -> Mux/3
  Mux2/1 -> ApplyRotation/1
  ApplyRotation/1 -> Mux/1
  Selector2/1 -> Mux4/3
  Selector1/1 -> Mux4/2
  Selector9/1 -> Mux4/1
  Selector17/1 -> Mux6/3
  Selector16/1 -> Mux6/2
  Selector18/1 -> Mux6/1
  Selector14/1 -> Mux5/3
  Selector13/1 -> Mux5/2
  Selector15/1 -> Mux5/1
  Selector11/1 -> Mux2/3
  Selector10/1 -> Mux2/2
  Selector12/1 -> Mux2/1
  Mux3/1 -> Selector8/1, Selector7/1, Selector3/1, Selector18/1, Selector16/1, Selector17/1, Selector6/1, Selector20/1, Selector19/1, Selector21/1, Selector5/1, Selector4/1, Selector14/1, Selector13/1, Selector15/1, Selector2/1, Selector1/1, Selector9/1, Selector12/1, Selector10/1, Selector11/1
  Mux1/1 -> Add2/2
  Constant/1 -> Mux1/2
  Add2/1 -> Traj2State2/1(traj)
  Selector/1 -> Mux3/2
  Traj Org/1 -> Mux3/1
  Offset/1 -> Mux1/1, Selector/1
  Mux/1 -> Add2/1
  Traj2State2/1(state) -> state/1

== system Experiment_06081908_cs/Audi_A8_Sedan_2/Trajectories/TrajCoGOffset ==
  State In : Inport
  Add : Sum  Inputs=+-+
  Add1 : Sum
  ApplyRotation : PreScanSimulinkLibrary/ApplyRotation  SystemSampleTime=-1  VariantActivationTime=update diagram  Latency=0  AutoFrameSizeCalculation=off
  ApplyRotation1 : PreScanSimulinkLibrary/ApplyRotation  SystemSampleTime=-1  VariantActivationTime=update diagram  Latency=0  AutoFrameSizeCalculation=off
  CoG Offset : Constant  Value=[0 0 CoGOffsetZ]
  Degrees to Radians : simulink_extras/Transformations/Degrees to Radians
  Demux1 : Demux  Outputs=[3 3 3]
  Mux : Mux  Inputs=[3 3 3]
  Orientation : Constant  Value=[InitRoll InitPitch 0]
  State Out : Outport
  wires:
  State In/1 -> Demux1/1
  Demux1/1 -> Add/1
  Add/1 -> Mux/1
  Demux1/3 -> Mux/3, Add1/2
  Mux/1 -> State Out/1
  Demux1/2 -> Mux/2
  Orientation/1 -> Degrees to Radians/1
  ApplyRotation/1 -> Add/3
  ApplyRotation1/1 -> Add/2
  Add1/1 -> ApplyRotation/2
  CoG Offset/1 -> ApplyRotation1/1, ApplyRotation/1
  Degrees to Radians/1 -> Add1/1, ApplyRotation1/2

== system Experiment_06081908_cs/Audi_A8_Sedan_2/Trajectories/Trajectory_1 ==
  From Workspace : FromWorkspace  VariableName=trajectory  SampleTime=TimeStep  ZeroCross=off  OutputAfterFinalValue=Holding final value
  From Workspace1 : FromWorkspace  VariableName=trajectory  SampleTime=TimeStep  ZeroCross=off  OutputAfterFinalValue=Setting to zero
  Mux : Mux  Inputs=2
  Selector1 : Selector  InputPortWidth=24  IndexOptions=Index vector (dialog)  Indices=[7:18]  OutputSizes=1
  Selector9 : Selector  InputPortWidth=24  IndexOptions=Index vector (dialog)  Indices=[1:6]  OutputSizes=1
  trajectory : Outport
  wires:
  From Workspace/1 -> Selector9/1
  From Workspace1/1 -> Selector1/1
  Mux/1 -> trajectory/1
  Selector9/1 -> Mux/1
  Selector1/1 -> Mux/2

== system Experiment_06081908_cs/Box_1/Dynamics_Empty/MuxState ==
  note: mode: Dynamics
  note: mode: Positioning
  note: mode: Dynamics
      | VelVEHICLE
      | wrt VEH
  note: AnglesVEHICLE
      | wrtGLOB
  note: For state mode 'Dynamic' positions
      | are not taken into account, as they
      | are computed by integrating velocity.
      | Click annotation for Help.
  x [m] : Inport  SampleTime=TimeStep
  y [m] : Inport  Port=2  SampleTime=TimeStep
  z [m] : Inport  Port=3  SampleTime=TimeStep
  dx [m/s] : Inport  Port=4  SampleTime=TimeStep
  dy [m/s] : Inport  Port=5  SampleTime=TimeStep
  dz [m/s] : Inport  Port=6  SampleTime=TimeStep
  R [rad] : Inport  Port=7  SampleTime=TimeStep
  P [rad] : Inport  Port=8  SampleTime=TimeStep
  Y [rad] : Inport  Port=9  SampleTime=TimeStep
  Constant : Constant  DisableCoverage=on  Value=positioningmode
  Discrete-Time Integrator : DiscreteIntegrator  SampleTime=TimeStep  ICPrevOutput=DiscIntNeverNeededParam  ICPrevScaledInput=DiscIntNeverNeededParam
  Ground : Ground
  Ground1 : Ground
  Mux1 : Mux  Inputs=[3 3]
  Mux2 : Mux  Inputs=3
  Mux3 : Mux  Inputs=3
  Mux4 : Mux  Inputs=3
  Mux5 : Mux  Inputs=[3 3]
  Mux6 : Mux  Inputs=[6 3]
  Switch : Switch  Threshold=0.5
  Transformation_BODY2GLOBAL : PreScanSimulinkLibrary/Simple_Vehicle_Dynamics/Chassis/MuxDynState/Transformation_BODY2GLOBAL  SystemSampleTime=-1  VariantActivationTime=update diagram  Latency=0  AutoFrameSizeCalculation=off
  mux3 : Mux  Inputs=3
  state : Outport
  wires:
  Constant/1 -> Switch/2
  Mux6/1 -> state/1
  Mux4/1 -> Mux1/1
  Mux5/1 -> Switch/3
  Mux1/1 -> Switch/1
  Switch/1 -> Mux6/1  "PosVeh wrt  GLOB"
  P [rad]/1 -> Mux3/2
  R [rad]/1 -> Mux3/1
  dz [m/s]/1 -> Mux2/3
  dy [m/s]/1 -> Mux2/2
  dx [m/s]/1 -> Mux2/1
  z [m]/1 -> Mux4/3
  y [m]/1 -> Mux4/2
  x [m]/1 -> Mux4/1
  Ground1/1 -> mux3/2  "pitch"
  Y [rad]/1 -> mux3/3, Mux3/3  "yaw"
  Mux3/1 -> Mux6/2
  Transformation_BODY2GLOBAL/1 -> Discrete-Time Integrator/1, Mux5/2  "VelVEH wrt  GLOB"
  mux3/1 -> Transformation_BODY2GLOBAL/2
  Ground/1 -> mux3/1  "roll"
  Mux2/1 -> Mux1/2, Transformation_BODY2GLOBAL/1
  Discrete-Time Integrator/1 -> Mux5/1  "PosVEH wrt  GLOB"

== system Experiment_06081908_cs/Box_1/SELF_Demux/compas converter ==
  rotz [rad] : Inport
  cart2compas : Subsystem
  rad2deg : Gain  Gain=180/pi
  heading [deg] : Outport
  wires:
  rad2deg/1 -> cart2compas/1(Angle [deg])
  rotz [rad]/1 -> rad2deg/1
  cart2compas/1(heading [deg]) -> heading [deg]/1

== system Experiment_06081908_cs/Box_2/Dynamics_Empty/MuxState ==
  note: mode: Dynamics
  note: mode: Positioning
  note: mode: Dynamics
      | VelVEHICLE
      | wrt VEH
  note: AnglesVEHICLE
      | wrtGLOB
  note: For state mode 'Dynamic' positions
      | are not taken into account, as they
      | are computed by integrating velocity.
      | Click annotation for Help.
  x [m] : Inport  SampleTime=TimeStep
  y [m] : Inport  Port=2  SampleTime=TimeStep
  z [m] : Inport  Port=3  SampleTime=TimeStep
  dx [m/s] : Inport  Port=4  SampleTime=TimeStep
  dy [m/s] : Inport  Port=5  SampleTime=TimeStep
  dz [m/s] : Inport  Port=6  SampleTime=TimeStep
  R [rad] : Inport  Port=7  SampleTime=TimeStep
  P [rad] : Inport  Port=8  SampleTime=TimeStep
  Y [rad] : Inport  Port=9  SampleTime=TimeStep
  Constant : Constant  DisableCoverage=on  Value=positioningmode
  Discrete-Time Integrator : DiscreteIntegrator  SampleTime=TimeStep  ICPrevOutput=DiscIntNeverNeededParam  ICPrevScaledInput=DiscIntNeverNeededParam
  Ground : Ground
  Ground1 : Ground
  Mux1 : Mux  Inputs=[3 3]
  Mux2 : Mux  Inputs=3
  Mux3 : Mux  Inputs=3
  Mux4 : Mux  Inputs=3
  Mux5 : Mux  Inputs=[3 3]
  Mux6 : Mux  Inputs=[6 3]
  Switch : Switch  Threshold=0.5
  Transformation_BODY2GLOBAL : PreScanSimulinkLibrary/Simple_Vehicle_Dynamics/Chassis/MuxDynState/Transformation_BODY2GLOBAL  SystemSampleTime=-1  VariantActivationTime=update diagram  Latency=0  AutoFrameSizeCalculation=off
  mux3 : Mux  Inputs=3
  state : Outport
  wires:
  Constant/1 -> Switch/2
  Mux6/1 -> state/1
  Mux4/1 -> Mux1/1
  Mux5/1 -> Switch/3
  Mux1/1 -> Switch/1
  Switch/1 -> Mux6/1  "PosVeh wrt  GLOB"
  P [rad]/1 -> Mux3/2
  R [rad]/1 -> Mux3/1
  dz [m/s]/1 -> Mux2/3
  dy [m/s]/1 -> Mux2/2
  dx [m/s]/1 -> Mux2/1
  z [m]/1 -> Mux4/3
  y [m]/1 -> Mux4/2
  x [m]/1 -> Mux4/1
  Ground1/1 -> mux3/2  "pitch"
  Y [rad]/1 -> mux3/3, Mux3/3  "yaw"
  Mux3/1 -> Mux6/2
  Transformation_BODY2GLOBAL/1 -> Discrete-Time Integrator/1, Mux5/2  "VelVEH wrt  GLOB"
  mux3/1 -> Transformation_BODY2GLOBAL/2
  Ground/1 -> mux3/1  "roll"
  Mux2/1 -> Mux1/2, Transformation_BODY2GLOBAL/1
  Discrete-Time Integrator/1 -> Mux5/1  "PosVEH wrt  GLOB"

== system Experiment_06081908_cs/Box_2/SELF_Demux/compas converter ==
  rotz [rad] : Inport
  cart2compas : Subsystem
  rad2deg : Gain  Gain=180/pi
  heading [deg] : Outport
  wires:
  rad2deg/1 -> cart2compas/1(Angle [deg])
  rotz [rad]/1 -> rad2deg/1
  cart2compas/1(heading [deg]) -> heading [deg]/1

== system Experiment_06081908_cs/Box_3/Dynamics_Empty/MuxState ==
  note: mode: Dynamics
  note: mode: Positioning
  note: mode: Dynamics
      | VelVEHICLE
      | wrt VEH
  note: AnglesVEHICLE
      | wrtGLOB
  note: For state mode 'Dynamic' positions
      | are not taken into account, as they
      | are computed by integrating velocity.
      | Click annotation for Help.
  x [m] : Inport  SampleTime=TimeStep
  y [m] : Inport  Port=2  SampleTime=TimeStep
  z [m] : Inport  Port=3  SampleTime=TimeStep
  dx [m/s] : Inport  Port=4  SampleTime=TimeStep
  dy [m/s] : Inport  Port=5  SampleTime=TimeStep
  dz [m/s] : Inport  Port=6  SampleTime=TimeStep
  R [rad] : Inport  Port=7  SampleTime=TimeStep
  P [rad] : Inport  Port=8  SampleTime=TimeStep
  Y [rad] : Inport  Port=9  SampleTime=TimeStep
  Constant : Constant  DisableCoverage=on  Value=positioningmode
  Discrete-Time Integrator : DiscreteIntegrator  SampleTime=TimeStep  ICPrevOutput=DiscIntNeverNeededParam  ICPrevScaledInput=DiscIntNeverNeededParam
  Ground : Ground
  Ground1 : Ground
  Mux1 : Mux  Inputs=[3 3]
  Mux2 : Mux  Inputs=3
  Mux3 : Mux  Inputs=3
  Mux4 : Mux  Inputs=3
  Mux5 : Mux  Inputs=[3 3]
  Mux6 : Mux  Inputs=[6 3]
  Switch : Switch  Threshold=0.5
  Transformation_BODY2GLOBAL : PreScanSimulinkLibrary/Simple_Vehicle_Dynamics/Chassis/MuxDynState/Transformation_BODY2GLOBAL  SystemSampleTime=-1  VariantActivationTime=update diagram  Latency=0  AutoFrameSizeCalculation=off
  mux3 : Mux  Inputs=3
  state : Outport
  wires:
  Constant/1 -> Switch/2
  Mux6/1 -> state/1
  Mux4/1 -> Mux1/1
  Mux5/1 -> Switch/3
  Mux1/1 -> Switch/1
  Switch/1 -> Mux6/1  "PosVeh wrt  GLOB"
  P [rad]/1 -> Mux3/2
  R [rad]/1 -> Mux3/1
  dz [m/s]/1 -> Mux2/3
  dy [m/s]/1 -> Mux2/2
  dx [m/s]/1 -> Mux2/1
  z [m]/1 -> Mux4/3
  y [m]/1 -> Mux4/2
  x [m]/1 -> Mux4/1
  Ground1/1 -> mux3/2  "pitch"
  Y [rad]/1 -> mux3/3, Mux3/3  "yaw"
  Mux3/1 -> Mux6/2
  Transformation_BODY2GLOBAL/1 -> Discrete-Time Integrator/1, Mux5/2  "VelVEH wrt  GLOB"
  mux3/1 -> Transformation_BODY2GLOBAL/2
  Ground/1 -> mux3/1  "roll"
  Mux2/1 -> Mux1/2, Transformation_BODY2GLOBAL/1
  Discrete-Time Integrator/1 -> Mux5/1  "PosVEH wrt  GLOB"

== system Experiment_06081908_cs/Box_3/SELF_Demux/compas converter ==
  rotz [rad] : Inport
  cart2compas : Subsystem
  rad2deg : Gain  Gain=180/pi
  heading [deg] : Outport
  wires:
  rad2deg/1 -> cart2compas/1(Angle [deg])
  rotz [rad]/1 -> rad2deg/1
  cart2compas/1(heading [deg]) -> heading [deg]/1

== system Experiment_06081908_cs/Box_4/Dynamics_Empty/MuxState ==
  note: mode: Dynamics
  note: mode: Positioning
  note: mode: Dynamics
      | VelVEHICLE
      | wrt VEH
  note: AnglesVEHICLE
      | wrtGLOB
  note: For state mode 'Dynamic' positions
      | are not taken into account, as they
      | are computed by integrating velocity.
      | Click annotation for Help.
  x [m] : Inport  SampleTime=TimeStep
  y [m] : Inport  Port=2  SampleTime=TimeStep
  z [m] : Inport  Port=3  SampleTime=TimeStep
  dx [m/s] : Inport  Port=4  SampleTime=TimeStep
  dy [m/s] : Inport  Port=5  SampleTime=TimeStep
  dz [m/s] : Inport  Port=6  SampleTime=TimeStep
  R [rad] : Inport  Port=7  SampleTime=TimeStep
  P [rad] : Inport  Port=8  SampleTime=TimeStep
  Y [rad] : Inport  Port=9  SampleTime=TimeStep
  Constant : Constant  DisableCoverage=on  Value=positioningmode
  Discrete-Time Integrator : DiscreteIntegrator  SampleTime=TimeStep  ICPrevOutput=DiscIntNeverNeededParam  ICPrevScaledInput=DiscIntNeverNeededParam
  Ground : Ground
  Ground1 : Ground
  Mux1 : Mux  Inputs=[3 3]
  Mux2 : Mux  Inputs=3
  Mux3 : Mux  Inputs=3
  Mux4 : Mux  Inputs=3
  Mux5 : Mux  Inputs=[3 3]
  Mux6 : Mux  Inputs=[6 3]
  Switch : Switch  Threshold=0.5
  Transformation_BODY2GLOBAL : PreScanSimulinkLibrary/Simple_Vehicle_Dynamics/Chassis/MuxDynState/Transformation_BODY2GLOBAL  SystemSampleTime=-1  VariantActivationTime=update diagram  Latency=0  AutoFrameSizeCalculation=off
  mux3 : Mux  Inputs=3
  state : Outport
  wires:
  Constant/1 -> Switch/2
  Mux6/1 -> state/1
  Mux4/1 -> Mux1/1
  Mux5/1 -> Switch/3
  Mux1/1 -> Switch/1
  Switch/1 -> Mux6/1  "PosVeh wrt  GLOB"
  P [rad]/1 -> Mux3/2
  R [rad]/1 -> Mux3/1
  dz [m/s]/1 -> Mux2/3
  dy [m/s]/1 -> Mux2/2
  dx [m/s]/1 -> Mux2/1
  z [m]/1 -> Mux4/3
  y [m]/1 -> Mux4/2
  x [m]/1 -> Mux4/1
  Ground1/1 -> mux3/2  "pitch"
  Y [rad]/1 -> mux3/3, Mux3/3  "yaw"
  Mux3/1 -> Mux6/2
  Transformation_BODY2GLOBAL/1 -> Discrete-Time Integrator/1, Mux5/2  "VelVEH wrt  GLOB"
  mux3/1 -> Transformation_BODY2GLOBAL/2
  Ground/1 -> mux3/1  "roll"
  Mux2/1 -> Mux1/2, Transformation_BODY2GLOBAL/1
  Discrete-Time Integrator/1 -> Mux5/1  "PosVEH wrt  GLOB"

== system Experiment_06081908_cs/Box_4/SELF_Demux/compas converter ==
  rotz [rad] : Inport
  cart2compas : Subsystem
  rad2deg : Gain  Gain=180/pi
  heading [deg] : Outport
  wires:
  rad2deg/1 -> cart2compas/1(Angle [deg])
  rotz [rad]/1 -> rad2deg/1
  cart2compas/1(heading [deg]) -> heading [deg]/1

== system Experiment_06081908_cs/Box_8/Dynamics_Empty/MuxState ==
  note: mode: Dynamics
  note: mode: Positioning
  note: mode: Dynamics
      | VelVEHICLE
      | wrt VEH
  note: AnglesVEHICLE
      | wrtGLOB
  note: For state mode 'Dynamic' positions
      | are not taken into account, as they
      | are computed by integrating velocity.
      | Click annotation for Help.
  x [m] : Inport  SampleTime=TimeStep
  y [m] : Inport  Port=2  SampleTime=TimeStep
  z [m] : Inport  Port=3  SampleTime=TimeStep
  dx [m/s] : Inport  Port=4  SampleTime=TimeStep
  dy [m/s] : Inport  Port=5  SampleTime=TimeStep
  dz [m/s] : Inport  Port=6  SampleTime=TimeStep
  R [rad] : Inport  Port=7  SampleTime=TimeStep
  P [rad] : Inport  Port=8  SampleTime=TimeStep
  Y [rad] : Inport  Port=9  SampleTime=TimeStep
  Constant : Constant  DisableCoverage=on  Value=positioningmode
  Discrete-Time Integrator : DiscreteIntegrator  SampleTime=TimeStep  ICPrevOutput=DiscIntNeverNeededParam  ICPrevScaledInput=DiscIntNeverNeededParam
  Ground : Ground
  Ground1 : Ground
  Mux1 : Mux  Inputs=[3 3]
  Mux2 : Mux  Inputs=3
  Mux3 : Mux  Inputs=3
  Mux4 : Mux  Inputs=3
  Mux5 : Mux  Inputs=[3 3]
  Mux6 : Mux  Inputs=[6 3]
  Switch : Switch  Threshold=0.5
  Transformation_BODY2GLOBAL : PreScanSimulinkLibrary/Simple_Vehicle_Dynamics/Chassis/MuxDynState/Transformation_BODY2GLOBAL  SystemSampleTime=-1  VariantActivationTime=update diagram  Latency=0  AutoFrameSizeCalculation=off
  mux3 : Mux  Inputs=3
  state : Outport
  wires:
  Constant/1 -> Switch/2
  Mux6/1 -> state/1
  Mux4/1 -> Mux1/1
  Mux5/1 -> Switch/3
  Mux1/1 -> Switch/1
  Switch/1 -> Mux6/1  "PosVeh wrt  GLOB"
  P [rad]/1 -> Mux3/2
  R [rad]/1 -> Mux3/1
  dz [m/s]/1 -> Mux2/3
  dy [m/s]/1 -> Mux2/2
  dx [m/s]/1 -> Mux2/1
  z [m]/1 -> Mux4/3
  y [m]/1 -> Mux4/2
  x [m]/1 -> Mux4/1
  Ground1/1 -> mux3/2  "pitch"
  Y [rad]/1 -> mux3/3, Mux3/3  "yaw"
  Mux3/1 -> Mux6/2
  Transformation_BODY2GLOBAL/1 -> Discrete-Time Integrator/1, Mux5/2  "VelVEH wrt  GLOB"
  mux3/1 -> Transformation_BODY2GLOBAL/2
  Ground/1 -> mux3/1  "roll"
  Mux2/1 -> Mux1/2, Transformation_BODY2GLOBAL/1
  Discrete-Time Integrator/1 -> Mux5/1  "PosVEH wrt  GLOB"

== system Experiment_06081908_cs/Box_8/SELF_Demux/compas converter ==
  rotz [rad] : Inport
  cart2compas : Subsystem
  rad2deg : Gain  Gain=180/pi
  heading [deg] : Outport
  wires:
  rad2deg/1 -> cart2compas/1(Angle [deg])
  rotz [rad]/1 -> rad2deg/1
  cart2compas/1(heading [deg]) -> heading [deg]/1

== system Experiment_06081908_cs/Audi_A8_Sedan_1/Dynamics_UserSpecified/CarSim2PreScanSTATE/Transformation_SprungMassCarSim2PreScan ==
  In1 : Inport
  Demux : Demux  Outputs=3
  Ini z-position VEHICLE wrt GLOBAL axis system [m] : Constant  Value=z0
  Mux : Mux  Inputs=3
  Sum1 : Sum  Inputs=+-
  Out1 : Outport
  wires:
  Mux/1 -> Out1/1
  Ini z-position VEHICLE wrt GLOBAL axis system [m]/1 -> Sum1/2
  Demux/1 -> Mux/1
  Sum1/1 -> Mux/3
  Demux/3 -> Sum1/1
  Demux/2 -> Mux/2
  In1/1 -> Demux/1

== system Experiment_06081908_cs/Audi_A8_Sedan_1/SELF_Demux/compas converter/cart2compas ==
  Angle [deg] : Inport
  Constant : Constant  Value=90
  Constant1 : Constant  Value=360
  Gain : Gain  Gain=1/360
  Gain1 : Gain  Gain=360
  Gain2 : Gain  Gain=-1
  Rounding Function : Rounding
  Sum : Sum  Inputs=|-+
  Sum1 : Sum  Inputs=-+|
  Sum2 : Sum  Inputs=++|
  heading [deg] : Outport
  wires:
  Gain/1 -> Rounding Function/1
  Rounding Function/1 -> Gain1/1
  Gain1/1 -> Sum/1
  Angle [deg]/1 -> Sum1/2
  Sum/1 -> Gain2/1
  Sum1/1 -> Gain/1, Sum/2
  Constant/1 -> Sum1/1
  Gain2/1 -> Sum2/2
  Constant1/1 -> Sum2/1
  Sum2/1 -> heading [deg]/1

== system Experiment_06081908_cs/Audi_A8_Sedan_1/control module1/control main/chassic steering system ==
  LQR_final_angle : Inport
  Constant : Constant  Value=la
  Constant1 : Constant  Value=lb
  Constant17 : Constant  Value=c_factor
  Divide : Product  Inputs=*/
  Gain3 : Gain  Gain=180/pi
  Gain4 : Gain  Gain=360
  MATLAB Function : MATLAB Function  TreatAsAtomicUnit=on
  Saturation : Saturate  UpperLimit=70  LowerLimit=-70
  Saturation1 : Saturate  UpperLimit=1.2217  LowerLimit=-1.2217
  transfer right wheel angle to rack displancement : Lookup_n-D  NumberOfTableDimensions=1  BreakpointsForDimension1=right_wheel_ground  Table=rack_displacement  InternalRulePriority=Speed  RndMeth=Simplest  InputSameDT=on
  lat_steer_sw[deg] : Outport
  wires:
  transfer right wheel angle to rack displancement/1 -> Divide/1
  Constant17/1 -> Divide/2
  Gain4/1 -> lat_steer_sw[deg]/1
  Divide/1 -> Gain4/1
  Saturation/1 -> transfer right wheel angle to rack displancement/1
  Constant/1 -> MATLAB Function/2(la)
  Gain3/1 -> Saturation/1
  Constant1/1 -> MATLAB Function/3(lb)
  LQR_final_angle/1 -> Saturation1/1
  Saturation1/1 -> MATLAB Function/1(u)
  MATLAB Function/1(right_steer) -> Gain3/1
